simulink model "Matrice_gravite_Gx"  (R2022b)
settings: Solver=VariableStepAuto  StartTime=0.0  StopTime=10.0  RelTol=1e-3
undefined symbols (not defined in the file): l1, l2, m1, m2
settings Model: Creator=cheye  LastModifiedBy=cheye

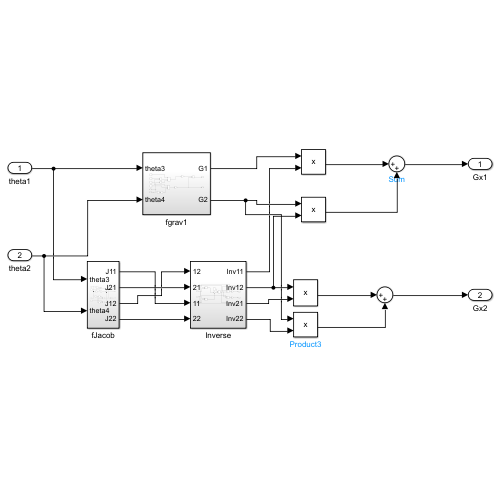
[thumbnail: Simulink's stored preview of the top-level diagram]
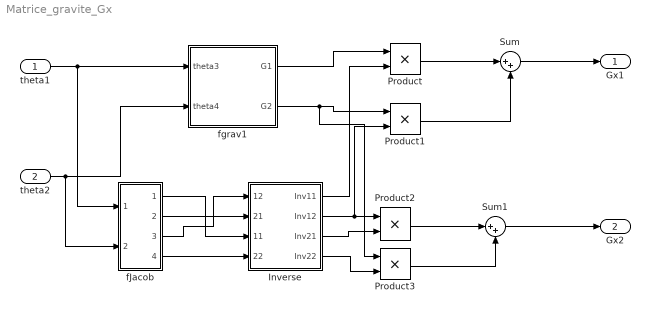
== system Matrice_gravite_Gx ==
  theta1 : Inport
  theta2 : Inport  Port=2
  Inverse : Subsystem
  Product{,1..3} (4 alike) : Product
  Sum : Sum  Inputs=|++
  Sum1 : Sum  Inputs=|++
  fJacob : Subsystem
  fgrav1 : Subsystem
  Gx1 : Outport
  Gx2 : Outport  Port=2
  wires:
  Sum1/1 -> Gx2/1
  theta1/1 -> fJacob/1(theta3), fgrav1/1(theta3)
  theta2/1 -> fJacob/2(theta4), fgrav1/2(theta4)
  fJacob/1(J11) -> Inverse/3(11)
  fJacob/2(J21) -> Inverse/2(21)
  fJacob/3(J12) -> Inverse/1(12)
  fJacob/4(J22) -> Inverse/4(22)
  Inverse/4(Inv22) -> Product3/2
  fgrav1/1(G1) -> Product/1
  fgrav1/2(G2) -> Product3/1, Product1/1
  Inverse/3(Inv21) -> Product2/2
  Inverse/2(Inv12) -> Product2/1, Product1/2
  Inverse/1(Inv11) -> Product/2
  Product/1 -> Sum/1
  Product1/1 -> Sum/2
  Product2/1 -> Sum1/1
  Product3/1 -> Sum1/2
  Sum/1 -> Gx1/1

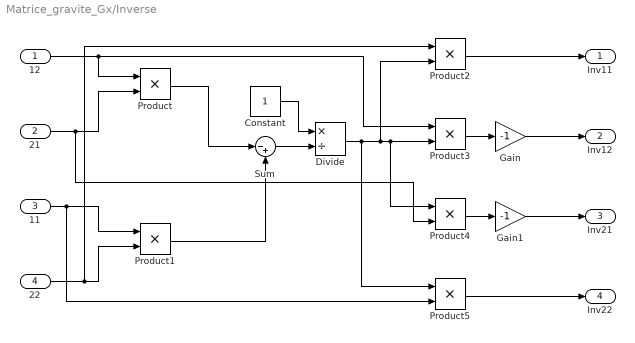
== system Matrice_gravite_Gx/Inverse ==
  12 : Inport
  21 : Inport  Port=2
  11 : Inport  Port=3
  22 : Inport  Port=4
  Constant : Constant
  Divide : Product  Inputs=*/
  Gain : Gain  Gain=-1
  Gain1 : Gain  Gain=-1
  Product{,1..5} (6 alike) : Product
  Sum : Sum  Inputs=|-+
  Inv11 : Outport
  Inv12 : Outport  Port=2
  Inv21 : Outport  Port=3
  Inv22 : Outport  Port=4
  wires:
  21/1 -> Product4/2, Product/2
  Product/1 -> Sum/1
  Divide/1 -> Product5/1, Product2/2, Product3/2, Product4/1
  22/1 -> Product1/2, Product2/1
  12/1 -> Product3/1, Product/1
  Product1/1 -> Sum/2
  11/1 -> Product5/2, Product1/1
  Constant/1 -> Divide/1
  Gain1/1 -> Inv21/1
  Product4/1 -> Gain1/1
  Product3/1 -> Gain/1
  Product5/1 -> Inv22/1
  Product2/1 -> Inv11/1
  Gain/1 -> Inv12/1
  Sum/1 -> Divide/2

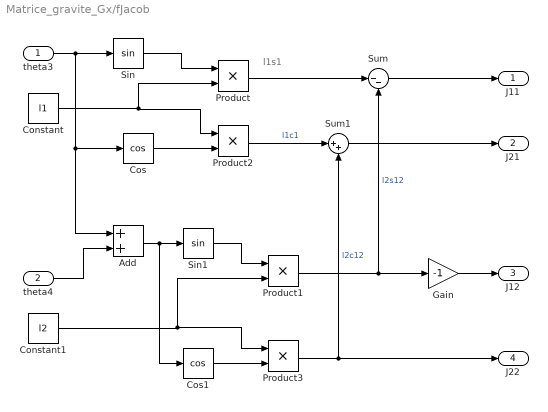
== system Matrice_gravite_Gx/fJacob ==
  note: l1s1
  theta3 : Inport
  theta4 : Inport  Port=2
  Add : Sum
  Constant : Constant  Value=l1
  Constant1 : Constant  Value=l2
  Cos : Trigonometry  Operator=cos
  Cos1 : Trigonometry  Operator=cos
  Gain : Gain  Gain=-1
  Product{,1..3} (4 alike) : Product
  Sin : Trigonometry
  Sin1 : Trigonometry
  Sum : Sum  Inputs=|--
  Sum1 : Sum  Inputs=|++
  J11 : Outport
  J21 : Outport  Port=2
  J12 : Outport  Port=3
  J22 : Outport  Port=4
  wires:
  theta4/1 -> Add/2
  Product3/1 -> J22/1, Sum1/2  "l2c12"
  Constant/1 -> Product/2, Product2/1
  Gain/1 -> J12/1
  Product2/1 -> Sum1/1  "l1c1"
  Add/1 -> Cos1/1, Sin1/1
  Product1/1 -> Sum/2, Gain/1  "l2s12"
  Product/1 -> Sum/1
  Cos/1 -> Product2/2
  Sin/1 -> Product/1
  theta3/1 -> Cos/1, Add/1, Sin/1
  Constant1/1 -> Product3/1, Product1/2
  Sum1/1 -> J21/1
  Sin1/1 -> Product1/1
  Cos1/1 -> Product3/2
  Sum/1 -> J11/1

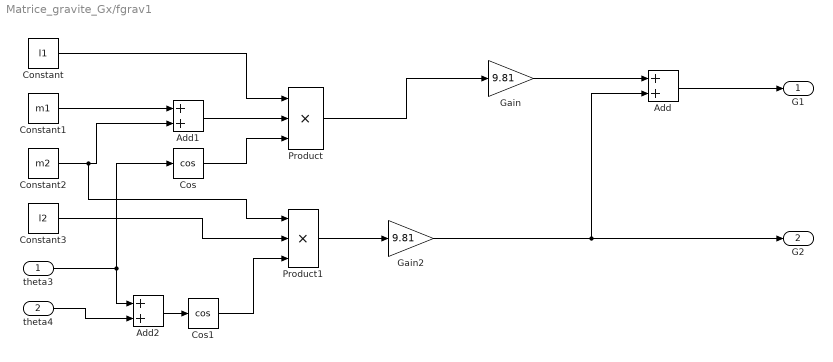
== system Matrice_gravite_Gx/fgrav1 ==
  theta3 : Inport
  theta4 : Inport  Port=2
  Add : Sum
  Add1 : Sum
  Add2 : Sum
  Constant : Constant  Value=l1
  Constant1 : Constant  Value=m1
  Constant2 : Constant  Value=m2
  Constant3 : Constant  Value=l2
  Cos : Trigonometry  Operator=cos
  Cos1 : Trigonometry  Operator=cos
  Gain : Gain  Gain=9.81
  Gain2 : Gain  Gain=9.81
  Product : Product  Inputs=3
  Product1 : Product  Inputs=3
  G1 : Outport
  G2 : Outport  Port=2
  wires:
  Add/1 -> G1/1
  Constant1/1 -> Add1/1
  Add2/1 -> Cos1/1
  Product/1 -> Gain/1
  Cos1/1 -> Product1/3
  Constant/1 -> Product/1
  Add1/1 -> Product/2
  Gain/1 -> Add/1
  Constant2/1 -> Product1/1, Add1/2
  Cos/1 -> Product/3
  theta4/1 -> Add2/2
  Gain2/1 -> G2/1, Add/2
  theta3/1 -> Cos/1, Add2/1
  Constant3/1 -> Product1/2
  Product1/1 -> Gain2/1
